simulink model "Mdl_Inverted_Pendulumn_Control"  (R2022b)
settings: Solver=ode23s  StartTime=0.0  StopTime=10  RelTol=1e-6  AbsTol=1e-6
values from neighbouring files (symbols this model uses):
  Lc = params.Lc    [B_PID_Design.m]    (also in C_Design.m = para.Lc)
  Lt = params.Lt    [B_PID_Design.m]    (also in C_Design.m = para.Lt)
undefined symbols (not defined in the file or in its folder): CtrlTs, DisAmp, DisPeriod, DisPhase, DisRatio, FedDcPoly, FedNcPoly, FwdDcPoly, FwdNcPoly, InitX, ModelSelFlag, NoisePara, SelFedSignalFlag, TFPara, Yd, YdStepTime
settings Model: Creator=User  LastModifiedBy=Administrator
settings SolverCC: AlgebraicLoopSolver=TrustRegion  AutoInsertRateTranBlk=on
settings DebuggingCC: SFMachineParentedDataDiag=warning  ArithmeticOperatorsInVariantConditions=warning
settings SFSimCC: CustomCodeUndefinedFunction=UseInterfaceOnly

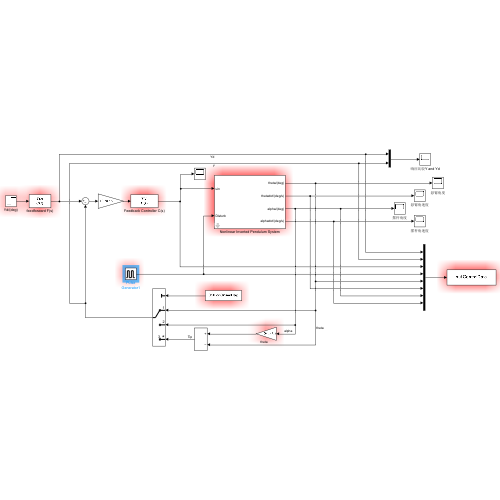
[thumbnail: Simulink's stored preview of the top-level diagram]
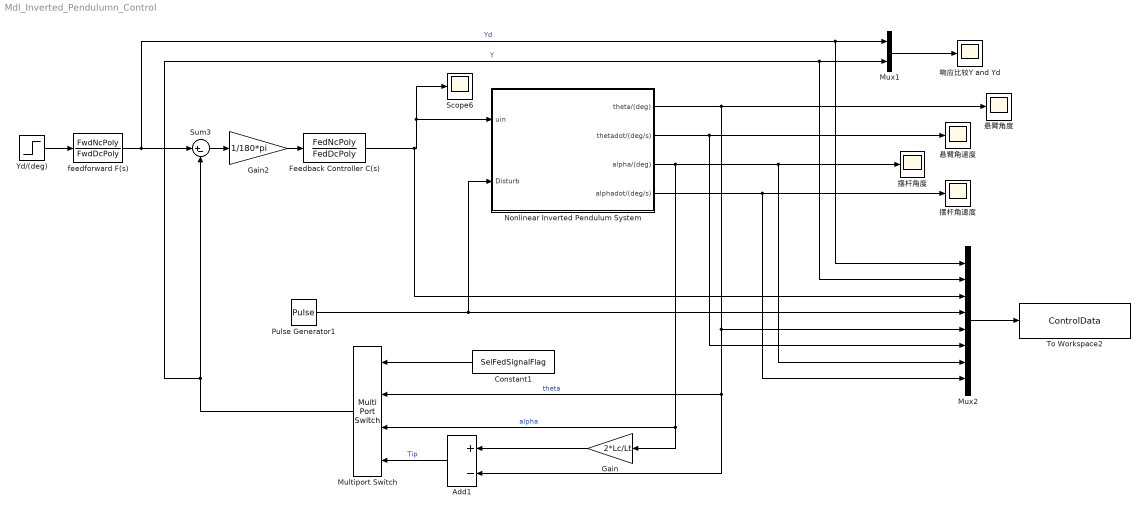
== system Mdl_Inverted_Pendulumn_Control ==
  Add1 : Sum  Inputs=+-
  Constant1 : Constant  Value=SelFedSignalFlag
  Feedback Controller C(s) : TransferFcn  Numerator=FedNcPoly  Denominator=FedDcPoly
  Gain : Gain  Gain=2*Lc/Lt
  Gain2 : Gain  Gain=1/180*pi
  Multiport Switch : MultiPortSwitch  SaturateOnIntegerOverflow=off  InputSameDT=off
  Mux1 : Mux  Inputs=2
  Mux2 : Mux  Inputs=8
  Nonlinear Inverted Pendulum System : Subsystem  mask{TFPara=TFPara, ModelSelFlag=ModelSelFlag, InitX=InitX, NoisePara=NoisePara}
  Pulse Generator1 : DiscretePulseGenerator  PulseType=Time based  Amplitude=DisAmp  Period=DisPeriod  PulseWidth=DisRatio  PhaseDelay=DisPhase
  Scope6 : Scope
  Sum3 : Sum  Inputs=|+-
  To Workspace2 : ToWorkspace  VariableName=ControlData  SaveFormat=Structure With Time  SampleTime=CtrlTs
  Yd/(deg) : Step  Time=YdStepTime  After=Yd  SampleTime=0
  feedforward F(s) : TransferFcn  Numerator=FwdNcPoly  Denominator=FwdDcPoly
  响应比较Y and Yd : Scope
  悬臂角度 : Scope
  悬臂角速度 : Scope
  摆杆角度 : Scope
  摆杆角速度 : Scope
  wires:
  Mux1/1 -> 响应比较Y and Yd/1
  Yd/(deg)/1 -> feedforward F(s)/1
  Nonlinear Inverted Pendulum System/2(thetadot/(deg/s)) -> Mux2/6, 悬臂角速度/1
  Feedback Controller C(s)/1 -> Mux2/3, Scope6/1, Nonlinear Inverted Pendulum System/1(uin)
  Nonlinear Inverted Pendulum System/4(alphadot/(deg/s)) -> Mux2/8, 摆杆角速度/1
  Mux2/1 -> To Workspace2/1
  Add1/1 -> Multiport Switch/4  "Tip"
  Nonlinear Inverted Pendulum System/3(alpha/(deg)) -> 摆杆角度/1, Mux2/7, Multiport Switch/3, Gain/1  "alpha"
  Nonlinear Inverted Pendulum System/1(theta/(deg)) -> 悬臂角度/1, Add1/2, Multiport Switch/2, Mux2/5  "theta"
  Constant1/1 -> Multiport Switch/1
  Multiport Switch/1 -> Sum3/2, Mux1/2, Mux2/2  "Y"
  Sum3/1 -> Gain2/1
  Gain2/1 -> Feedback Controller C(s)/1
  feedforward F(s)/1 -> Sum3/1, Mux1/1, Mux2/1  "Yd"
  Pulse Generator1/1 -> Nonlinear Inverted Pendulum System/2(Disturb), Mux2/4
  Gain/1 -> Add1/1

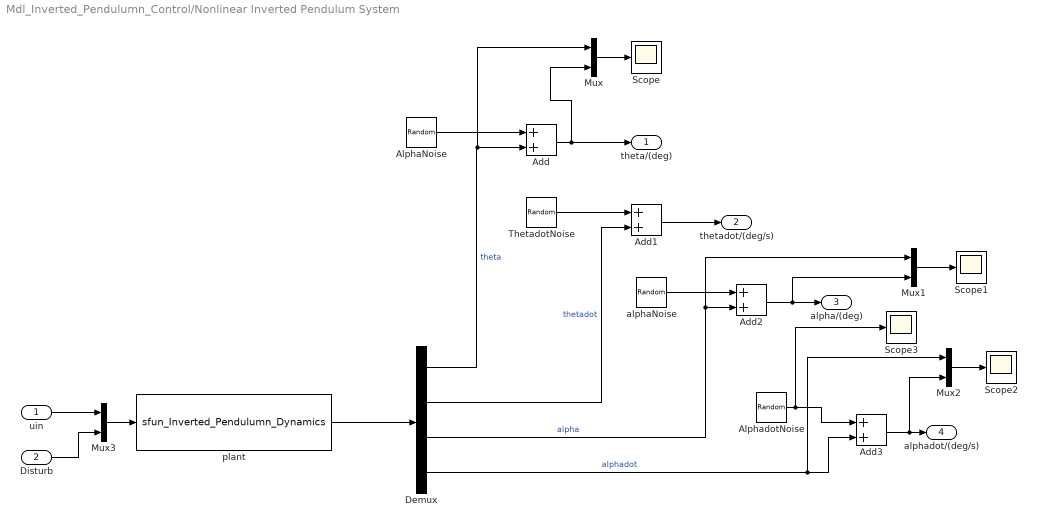
== system Mdl_Inverted_Pendulumn_Control/Nonlinear Inverted Pendulum System ==
  uin : Inport
  Disturb : Inport  Port=2
  Add{,1..3} (4 alike) : Sum
  AlphaNoise : RandomNumber  Mean=NoisePara(1,1)  Variance=NoisePara(1,2)  Seed=NoisePara(1,3)  SampleTime=NoisePara(1,4)
  AlphadotNoise : RandomNumber  Mean=NoisePara(4,1)  Variance=NoisePara(4,2)  Seed=NoisePara(4,3)  SampleTime=NoisePara(4,4)
  Demux : Demux
  Mux{,1..3} (4 alike) : Mux  Inputs=2
  Scope{,1..3} (4 alike) : Scope
  ThetadotNoise : RandomNumber  Mean=NoisePara(2,1)  Variance=NoisePara(2,2)  Seed=NoisePara(2,3)  SampleTime=NoisePara(2,4)
  alphaNoise : RandomNumber  Mean=NoisePara(3,1)  Variance=NoisePara(3,2)  Seed=NoisePara(3,3)  SampleTime=NoisePara(3,4)
  plant : S-Function  FunctionName=sfun_Inverted_Pendulumn_Dynamics  Parameters=InitX,TFPara,ModelSelFlag  SFunctionDeploymentMode=off  EnableBusSupport=off
  theta/(deg) : Outport
  thetadot/(deg/s) : Outport  Port=2
  alpha/(deg) : Outport  Port=3
  alphadot/(deg/s) : Outport  Port=4
  wires:
  Demux/4 -> Mux2/1, Add3/2  "alphadot"
  Demux/3 -> Mux1/1, Add2/2  "alpha"
  Demux/2 -> Add1/2  "thetadot"
  Demux/1 -> Mux/1, Add/2  "theta"
  AlphaNoise/1 -> Add/1
  Add/1 -> Mux/2, theta/(deg)/1
  ThetadotNoise/1 -> Add1/1
  Add1/1 -> thetadot/(deg/s)/1
  alphaNoise/1 -> Add2/1
  Add2/1 -> alpha/(deg)/1, Mux1/2
  AlphadotNoise/1 -> Scope3/1, Add3/1
  Add3/1 -> Mux2/2, alphadot/(deg/s)/1
  plant/1 -> Demux/1
  Mux/1 -> Scope/1
  Mux1/1 -> Scope1/1
  Mux2/1 -> Scope2/1
  Mux3/1 -> plant/1
  uin/1 -> Mux3/1
  Disturb/1 -> Mux3/2
